simulink model "queue_populator_modeling"  (R2020b)
settings: Solver=FixedStepDiscrete  StartTime=0.0  StopTime=10.0  FixedStep=0.1  RelTol=1e-3
undefined symbols (not defined in the file or in its folder): test_input
settings Model: Creator=rsub  LastModifiedBy=rsub

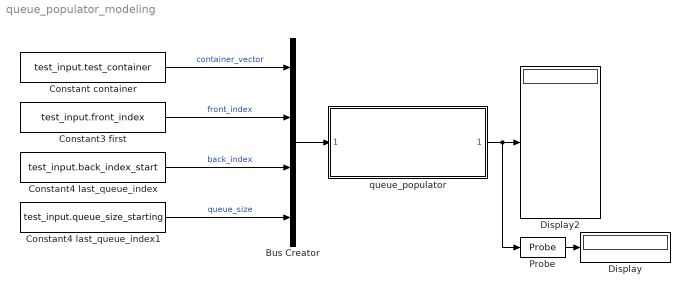
== system queue_populator_modeling ==
  Bus Creator : BusCreator  Inputs=4
  Constant container : Constant  Value=test_input.test_container
  Constant3 first : Constant  Value=test_input.front_index
  Constant4 last_queue_index : Constant  Value=test_input.back_index_start
  Constant4 last_queue_index1 : Constant  Value=test_input.queue_size_starting
  Display : Display
  Display2 : Display
  Probe : Probe  ProbeWidth=off  ProbeSampleTime=off  ProbeComplexSignal=off  ProbeSignalDimensions=on
  queue_populator : Subsystem  ReferencedSubsystem=queue_populator_model
  wires:
  queue_populator/1 -> Probe/1, Display2/1
  Constant container/1 -> Bus Creator/1  "container_vector"
  Bus Creator/1 -> queue_populator/1
  Constant3 first/1 -> Bus Creator/2  "front_index"
  Constant4 last_queue_index/1 -> Bus Creator/3  "back_index"
  Constant4 last_queue_index1/1 -> Bus Creator/4  "queue_size"
  Probe/1 -> Display/1
